simulink model "MPC"  (R2023a)
settings: Solver=VariableStepAuto  StartTime=0.0  StopTime=50  RelTol=1e-3
settings Model: Creator=belov  LastModifiedBy=belov

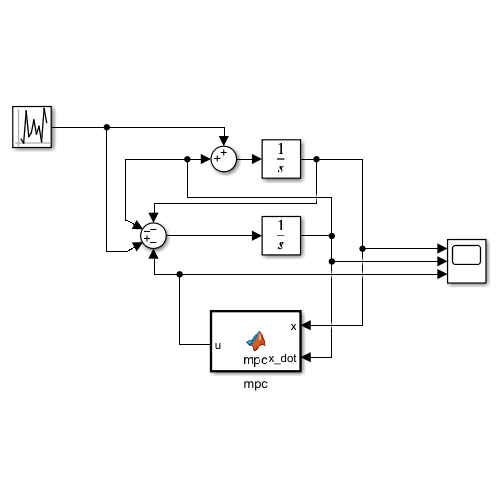
[thumbnail: Simulink's stored preview of the top-level diagram]
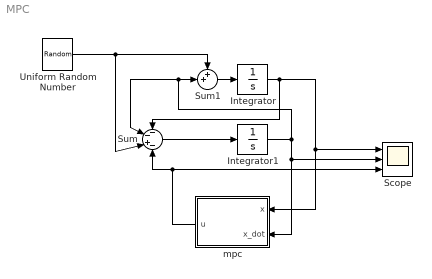
== system MPC ==
  Integrator : Integrator  InitialCondition=1
  Integrator1 : Integrator  InitialCondition=-1
  Scope : Scope  NumInputPorts=3
  Sum : Sum  Inputs=--+-
  Sum1 : Sum  Inputs=++|
  Uniform Random Number : UniformRandomNumber  Minimum=-0.05  Maximum=0.05  SampleTime=0.1
  mpc : MATLAB Function  TreatAsAtomicUnit=on
  wires:
  Integrator1/1 -> Scope/2, mpc/2(x_dot), Sum1/2, Sum/2
  Sum/1 -> Integrator1/1
  Integrator/1 -> mpc/1(x), Scope/1, Sum/1
  mpc/1(u) -> Sum/4, Scope/3
  Sum1/1 -> Integrator/1
  Uniform Random Number/1 -> Sum/3, Sum1/1

== matlab function MPC/mpc ==
  data: x input; u output; x_dot input
function u = mpc(x, x_dot)
x_k = [x; x_dot];
A = [0 1; -1 -1];
B = [0; 1];
Q = diag([100, 10]);
R = diag([10]);
N = 2;
n=size(A,1);
p=size(B,2);
M=[eye(n);zeros(N*n,n)];
C=zeros((N+1)*n,N*p);
tmp=eye(n);
for i=1:N
    rows =i*n+(1:n); 
    C(rows,:)=[tmp*B,C(rows-n, 1:end-p)];
    tmp= A*tmp;
    M(rows,:)=tmp;
end
% 定义Q_bar和R_bar
Q_bar = kron(eye(N),Q);
Q_bar = blkdiag(Q_bar,Q);
R_bar = kron(eye(N),R);
% 计算G, E, H
G = M'*Q_bar*M;
E = C'*Q_bar*M;
H = C'*Q_bar*C+R_bar;

U_k = zeros(N*p,1);
opts = optimoptions('quadprog','Algorithm','active-set');
U_k = quadprog(H, E * x_k, [], [], [], [], [], [], zeros(size(H, 1), 1), opts);
u = U_k(1, 1);
end
